simulink model "model2v2"  (R2020b)
settings: Solver=VariableStepAuto  StartTime=0.0  StopTime=10.0  RelTol=1e-3
settings Model: Creator=dkravchenko  LastModifiedBy=dkravchenko

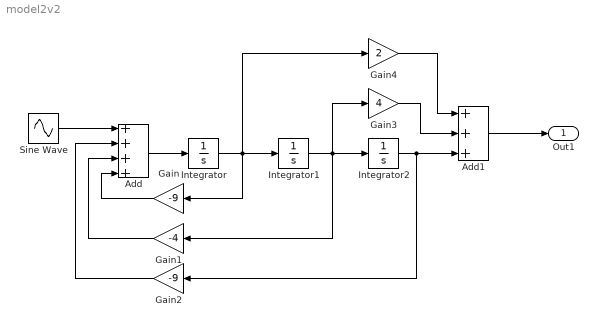
== system model2v2 ==
  Add : Sum  Inputs=++++
  Add1 : Sum  Inputs=+++
  Gain : Gain  Gain=-9
  Gain1 : Gain  Gain=-4
  Gain2 : Gain  Gain=-9
  Gain3 : Gain  Gain=4
  Gain4 : Gain  Gain=2
  Integrator : Integrator
  Integrator1 : Integrator
  Integrator2 : Integrator
  Sine Wave : Sin  Amplitude=0  Bias=1  SampleTime=0
  Out1 : Outport
  wires:
  Sine Wave/1 -> Add/1
  Add/1 -> Integrator/1
  Integrator/1 -> Gain4/1, Integrator1/1, Gain/1
  Gain/1 -> Add/4
  Integrator1/1 -> Gain3/1, Integrator2/1, Gain1/1
  Gain1/1 -> Add/3
  Integrator2/1 -> Add1/3, Gain2/1
  Gain2/1 -> Add/2
  Add1/1 -> Out1/1
  Gain3/1 -> Add1/2
  Gain4/1 -> Add1/1
